simulink model "TRN_KAISIM"  (R2022a)
settings: Solver=FixedStepAuto  StartTime=0.0  StopTime=300  FixedStep=0.04  RelTol=1e-3
PreLoadFcn:
  | load('BusStructureTRNsensor.mat');
  | load('BusStructureTRN.mat');
InitFcn:
  | load('BusStructureTRNsensor.mat');
  | load('BusStructureTRN.mat');
undefined symbols (not defined in the file or in its folder): Altitude_INS, Latitude_INS, Longitude_INS, residual, Result_Prev, TimeTag_Prev, TRN, TRNlib
libraries: simulink_extras x18, sharedtransform x3
(part 4 of 4)

== matlab function TRN_KAISIM/TRN/ModeManagementCSU/TrackingCSU/TrackingCSU_20230430/TrackingCSU_EKFupdate1/EKFUpdate_GPSinvalid/EKFUpdate_Update_GPSinvalid ==
  data: I input; xu_GPSinvalid output; P_GPSinvalid output; xp input; Pp input; latINSErrTRN_GPSinvalid output; lonINSErrTRN_GPSinvalid output; altINSErrTRN_GPSinvalid output; K input; Zmat_GPSinvalid input; Hmat_GPSinvalid input; Rmat_GPSinvalid input; xu_prev_GPSinvalid input; TimeTag_Prev input; hUncertainty_GPSinvalid output; vUncertainty_GPSinvalid output
function [xu_GPSinvalid, P_GPSinvalid, latINSErrTRN_GPSinvalid, lonINSErrTRN_GPSinvalid, altINSErrTRN_GPSinvalid, hUncertainty_GPSinvalid, vUncertainty_GPSinvalid] ...
    = EKFUpdate_Update_GPSinvalid(I, xp, Pp, K, Zmat_GPSinvalid, Hmat_GPSinvalid, Rmat_GPSinvalid, xu_prev_GPSinvalid, TimeTag_Prev)

xu_GPSinvalid = xp + K * (Zmat_GPSinvalid - Hmat_GPSinvalid*xp);
P_GPSinvalid = (I - K*Hmat_GPSinvalid) * Pp * (I - K*Hmat_GPSinvalid)' + K*Rmat_GPSinvalid*K';

hUncertainty_GPSinvalid = sqrt(abs(P_GPSinvalid(7,7) + P_GPSinvalid(8,8))) * 6378000;    % unit m
vUncertainty_GPSinvalid = sqrt(abs(P_GPSinvalid(9,9)));                       % unit m

latINSErrTRN_GPSinvalid = xu_GPSinvalid(7);
lonINSErrTRN_GPSinvalid = xu_GPSinvalid(8);
altINSErrTRN_GPSinvalid = xu_GPSinvalid(9);

if (TimeTag_Prev(6) == 1)
    xu_GPSinvalid = xu_prev_GPSinvalid;
    latINSErrTRN_GPSinvalid = xu_GPSinvalid(7);
    lonINSErrTRN_GPSinvalid = xu_GPSinvalid(8);
    altINSErrTRN_GPSinvalid = xu_GPSinvalid(9);
end

== matlab function TRN_KAISIM/TRN/TRN_visualization/MATLAB Function ==
  data: TRN_valid input; TRNOperatingEnv_Flag output; roll input; pitch input; INSDataNotvalid input
function TRNOperatingEnv_Flag  = TRNCorrCheck(TRN_valid, roll, pitch, INSDataNotvalid)

if (TRN_valid == true) && (abs(roll) < 15) && (abs(pitch) < 15) && (INSDataNotvalid == false)
    TRNOperatingEnv_Flag = boolean(true);
else
    TRNOperatingEnv_Flag = boolean(false);
end


end

== matlab function TRN_KAISIM/TRN/ModeManagementCSU/CorrelationValid/CorrelationValid function ==
  data: posUpdate input; MAD input; profileCnt input; TRNEstOfINSLatitudeErr output; TRNEstOfINSLongitudeErr output; TRNEstOfINSAltitudeErr output; GPSDataNotValid input; profileCnt output; NavigationMode output; AircraftPositionCorrectionValid output
function [TRNEstOfINSLatitudeErr, TRNEstOfINSLongitudeErr, TRNEstOfINSAltitudeErr, profileCnt, NavigationMode, AircraftPositionCorrectionValid] = CorrelationValid(posUpdate, MAD, profileCnt, GPSDataNotValid)

if (MAD < 50 && profileCnt >= 20) || ...
 (GPSDataNotValid == false && MAD < 50 && profileCnt >= 5)
    TRNEstOfINSLatitudeErr = -posUpdate(1) * 180/pi;
    TRNEstOfINSLongitudeErr = -posUpdate(2) * 180/pi;
    TRNEstOfINSAltitudeErr = 0.0;
    profileCnt = uint32(0);
    NavigationMode = false;
    AircraftPositionCorrectionValid = true;
else
    TRNEstOfINSLatitudeErr = 0.0;
    TRNEstOfINSLongitudeErr = 0.0;
    TRNEstOfINSAltitudeErr = 0.0;
    NavigationMode = true;
    AircraftPositionCorrectionValid = false;
end
end

== matlab function TRN_KAISIM/TRN/ModeManagementCSU/TrackingCSU/TrackingCSU_20230430/TrackingCSU_EKFupdate1/EKFUpdate_GPSvalid/EKFUpdate_Kgain_GPSvalid ==
  data: Hmat_GPSvalid input; Rmat_GPSvalid input; Pp input; K output
function K = EKFUpdate_Kgain_GPSvalid( Hmat_GPSvalid, Rmat_GPSvalid, Pp)


K = (Pp * Hmat_GPSvalid')/(Rmat_GPSvalid + Hmat_GPSvalid * Pp * Hmat_GPSvalid');




end

== matlab function TRN_KAISIM/TRN/ModeManagementCSU/TrackingCSU/TrackingCSU_20230430/TrackingCSU_EKFupdate1/EKFUpdate_GPSvalid/EKFUpdate_Predict_GPSvalid ==
  data: I output; xp output; Pp output; Fmatrix input; Gmatrix input; P input; Q input; dt input; Zmat_GPSvalid input; residual_GPSvalid output
function [I, xp, Pp, residual_GPSvalid] ...
    = EKFUpdate_Predict_GPSvalid(Fmatrix, Gmatrix, P, Q, dt, Zmat_GPSvalid)

x = zeros(15,1);
I = eye(max(size(Fmatrix)));

A = I + (Fmatrix*dt);
Q = (A*Gmatrix * Q * Gmatrix'*A') .* dt;

%-------------------------------------%
% Predicts states & covariance matrix
%-------------------------------------%
xp = A * x;
Pp = (A * P * A') + Q;
residual_GPSvalid = Zmat_GPSvalid(3);

end

== matlab function TRN_KAISIM/TRN/ModeManagementCSU/TrackingCSU/TrackingCSU_20230430/TrackingCSU_ConvertInput1/GPSflagcheck ==
  data: FoM input; GPSflag output; GPSDataNotValid input; AccY input
function GPSflag  = GPScheck(FoM, GPSDataNotValid, AccY)

GPSflag = uint32(2);

if GPSDataNotValid == 0
%     if EstHorErr < 100 && EstVerErr < 25 && state == 5
        if FoM <= 4
            GPSflag = uint32(1);
            if FoM <= 2 && abs(AccY) < 2
                GPSflag = uint32(0);
            end
        end
%    end
else
    GPSflag = uint32(2);
end

== matlab function TRN_KAISIM/TRN/ModeManagementCSU/TrackingCSU/TrackingCSU_20230430/TrackingCSU_EKFupdate1/EKFUpdate_GPSvalid/EKFUpdate_Update_GPSvalid ==
  data: I input; xu_GPSvalid output; P_GPSvalid output; xp input; Pp input; latINSErrTRN_GPSvalid output; lonINSErrTRN_GPSvalid output; altINSErrTRN_GPSvalid output; K input; Zmat_GPSvalid input; Hmat_GPSvalid input; Rmat_GPSvalid input; xu_prev_GPSvalid input; TimeTag_Prev input; hUncertainty_GPSvalid output; vUncertainty_GPSvalid output; GPSHorUncert input; GPSVerUncert input
function [xu_GPSvalid, P_GPSvalid, latINSErrTRN_GPSvalid, lonINSErrTRN_GPSvalid, altINSErrTRN_GPSvalid, hUncertainty_GPSvalid, vUncertainty_GPSvalid] ...
    = EKFUpdate_Update_GPSvalid(I, xp, Pp, K, Zmat_GPSvalid, Hmat_GPSvalid, Rmat_GPSvalid, xu_prev_GPSvalid, TimeTag_Prev, GPSHorUncert, GPSVerUncert)

xu_GPSvalid = xp + K * (Zmat_GPSvalid - Hmat_GPSvalid*xp);
P_GPSvalid = (I - K*Hmat_GPSvalid) * Pp * (I - K*Hmat_GPSvalid)' + K*Rmat_GPSvalid*K';

hUncertainty_GPSvalid = double(GPSHorUncert);     % unit m
vUncertainty_GPSvalid = double(GPSVerUncert);     % unit m


%---------------------------%
% Updates covariance matrix
%---------------------------%
% P = (I - K*H) * Pp * (I - K*H)' + K*R*K';

latINSErrTRN_GPSvalid = xu_GPSvalid(7);
lonINSErrTRN_GPSvalid = xu_GPSvalid(8);
altINSErrTRN_GPSvalid = xu_GPSvalid(9);
if (TimeTag_Prev(4) == 1)
    xu_GPSvalid = xu_prev_GPSvalid;
    latINSErrTRN_GPSvalid = xu_GPSvalid(7);
    lonINSErrTRN_GPSvalid = xu_GPSvalid(8);
    altINSErrTRN_GPSvalid = xu_GPSvalid(9);
end
%--------------------------------------------------------%

== matlab function TRN_KAISIM/TRN/ModeManagementCSU/TrackingCSU/TrackingCSU_20230430/Earth_radius ==
  data: M output; N output; Latitude_INS input; psi output
function [M, N, psi] = Earth_radius(Latitude_INS)

    a   = 6378137;          % Earth's equatorial radius
    b   = 6356752.314245;   % Earth's polar radius
    psi = Latitude_INS;     % psi(latitude_INS)
    M   = ((a*b)^2) / ( ( (a*cos(psi))^2 + (b*sin(psi))^2 )^(3/2) );    % radius  of  curvature  in  meridian
    N   = (a^2) / ( ( (a*cos(psi))^2 + (b*sin(psi))^2 )^(1/2) );        % radius  of  curvature  in  prime  vertical

end

== matlab function TRN_KAISIM/TRN/ModeManagementCSU/TrackingCSU/TrackingCSU_20230430/INS_Update_1553falt ==
  data: latINS input; latINS output; lonINS input; altINS input; velN input; velE input; velD input; TimeTag input; lonINS output; altINS output; dt input
function [latINS, lonINS, altINS] = INS_Update_1553falt(latINS, lonINS, altINS, velN, velE, velD, TimeTag, dt)

R0 = 6378000;

if TimeTag(5) == 1
    latINS = latINS + (velN * dt) * 1/(R0+altINS);
    lonINS = lonINS + (velE * dt) * 1/(R0+altINS);
    altINS = altINS + (velD * dt) * 1/(R0+altINS);
end

== matlab function TRN_KAISIM/TRN/ModeManagementCSU/TrackingCSU/TrackingCSU_20230430/TrackingCSU_EKFupdate1/MATLAB Function2 ==
  data: P_GPSinvalid input; Pmat_GPSvalid output; Pmat_GPSinvalid output; P_GPSvalid input; Weight_GPSvalid output; Weight_GPSinvalid output
function [Pmat_GPSvalid, Pmat_GPSinvalid, Weight_GPSvalid, Weight_GPSinvalid] = fcn(P_GPSinvalid, P_GPSvalid)

Pmat_GPSvalid = zeros(1,3);
Pmat_GPSinvalid = zeros(1,3);
Weight_GPSvalid = zeros(1,3);
Weight_GPSinvalid = zeros(1,3);

for i = 7:8

    Pmat_GPSvalid(1,i-6)   = sqrt(P_GPSvalid(i,i)) * 6378000;
    Pmat_GPSinvalid(1,i-6) = sqrt(P_GPSinvalid(i,i)) * 6378000;

end

Pmat_GPSvalid(1,3)   = sqrt(P_GPSvalid(9,9));
Pmat_GPSinvalid(1,3) = sqrt(P_GPSinvalid(9,9));

for j = 1:3
    Weight_GPSvalid(j)   = Pmat_GPSinvalid(1,j) / (Pmat_GPSvalid(1,j) + Pmat_GPSinvalid(1,j));  % Pmat이 클수록 못믿음
    Weight_GPSinvalid(j) = 1 - Weight_GPSvalid(j);
end

== matlab function TRN_KAISIM/TRN/TRN_visualization/Subsystem7/MATLAB Function ==
  data: Err_Lat_INS output; Err_Lon_INS output; Err_Alt_INS output; Err_Lat_GPS output; Err_Lon_GPS output; Err_Alt_GPS output; lat_Ref input; lon_Ref input; alt_Ref input; lat_INS input; lon_INS input; alt_INS input; Lat_INS output; Lon_INS output; Alt_INS output; Lat_Ref output; Lon_Ref output; Alt_Ref output; Lat_GPS input; Lon_GPS input; Alt_GPS input
function [Err_Lat_INS, Err_Lon_INS, Err_Alt_INS, Err_Lat_GPS, Err_Lon_GPS, Err_Alt_GPS,Lat_INS, Lon_INS, Alt_INS, Lat_Ref, Lon_Ref, Alt_Ref] = fcn(lat_Ref, lon_Ref, alt_Ref, lat_INS, lon_INS, alt_INS, Lat_GPS, Lon_GPS, Alt_GPS)

%% parameters
lat2m = 110961.7060516;
lon2m = 89476.51124;

%% setting

Lat_INS = lat_INS;               % INS Latitude
Lon_INS = lon_INS;               % INS Longitude
% Alt_INS = uint16(alt_INS);               % INS Altitude
Alt_INS = alt_INS;               % INS Altitude

Lat_Ref = lat_Ref;             % Ref Latitude
Lon_Ref = lon_Ref;             % Ref Longitude
% Alt_Ref = uint16(alt_Ref);             % Ref Altitude
Alt_Ref = alt_Ref;             % Ref Altitude

Err_Lat_INS = (Lat_Ref-Lat_INS)*lat2m;
Err_Lon_INS = (Lon_Ref-Lon_INS)*lon2m;
Err_Alt_INS = (Alt_Ref-Alt_INS);

Err_Lat_GPS = (Lat_Ref-Lat_GPS)*lat2m;
Err_Lon_GPS = (Lon_Ref-Lon_GPS)*lon2m;
Err_Alt_GPS = (Alt_Ref-Alt_GPS);

end
